simulink model "sampleModel153"  (R2021b)
settings: Solver=VariableStepAuto  StartTime=0.0  StopTime=10.0  RelTol=1e-3
undefined symbols (not defined in the file or in its folder): DiscIntNeverNeededParam
libraries: simulink x18, slpidlib x3
settings Model: Creator=user  LastModifiedBy=user

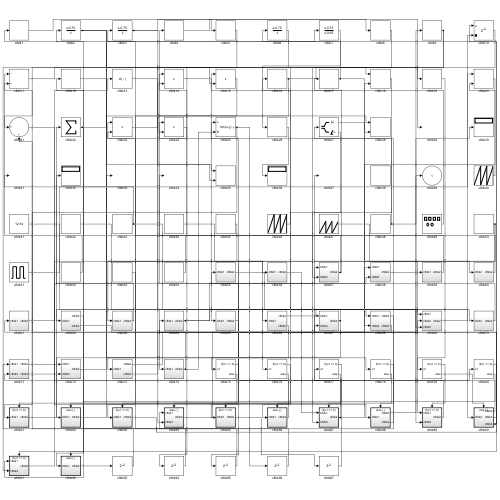
[thumbnail: Simulink's stored preview of the top-level diagram]
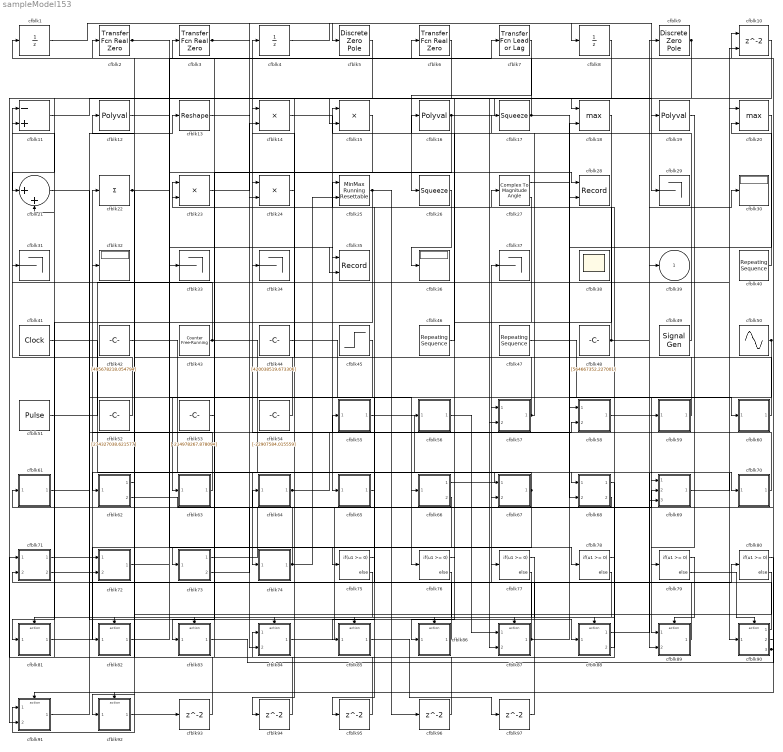
== system sampleModel153 ==
  cfblk1 : UnitDelay  HasFrameUpgradeWarning=on
  cfblk10 : Delay  ShowEnablePort=on  SampleTime=1
      settings: InputPortMap=u0,e6
  cfblk11 : Sum  Inputs=-+
  cfblk12 : Polyval  Coefs=[ +2.081618890e-019, -1.441693666e-014, +4.719686976e-010, -8.536869453e-006, +1.621573104e-001, -8.087801117e+001 ]
  cfblk13 : Reshape
  cfblk14 : Product
  cfblk15 : Product
  cfblk16 : Polyval  Coefs=[ +2.081618890e-019, -1.441693666e-014, +4.719686976e-010, -8.536869453e-006, +1.621573104e-001, -8.087801117e+001 ]
  cfblk17 : Squeeze
  cfblk18 : MinMax  Function=max  Inputs=2
  cfblk19 : Polyval  Coefs=[ +2.081618890e-019, -1.441693666e-014, +4.719686976e-010, -8.536869453e-006, +1.621573104e-001, -8.087801117e+001 ]
  cfblk2 : simulink/Discrete/Transfer Fcn Real Zero  ZeroZ=0.75  ICPrevInput=0.0  DoSatur=off
      settings: SourceProductBaseCode=SL
  cfblk20 : MinMax  Function=max  Inputs=2
  cfblk21 : Sum  Inputs=|++
  cfblk22 : Sum  Inputs=+
  cfblk23 : Product  Inputs=**
  cfblk24 : Product
  cfblk25 : simulink/Math Operations/MinMax Running Resettable  Function=min  vinit=0.0
  cfblk26 : Squeeze
  cfblk27 : ComplexToMagnitudeAngle
  cfblk28 : Record  FileSettingsInternal="{\"entries\":[{\"content\":{\"excelSettings\":{\"content\":{},\"type\":\"Streamout.ExcelSettings\"}},\"type\":\"Streamout.FileSettingStorage\",\"uuid\":\"2c212456-ffd4-42f7-90f6-1e0b846be94d\"}],\"packageUris\":[\"http://schema.mathworks.com/mf0/streamout_blocks/R2020a\"],\"version\":\"1.0\"}"  Layout=[1 1]  SignalsInternal="{\"entries\":[{\"content\":{\"signals\":[{\"content\":{\"blockPath\":[\"sampleModel153/cfblk28\"],\"channel\":[],\"dimensions\":[1],\"domain\":\"sampleModel153/cfblk28\",\"lineColor\":\"#a2142f\",\"plots\":[1],\"port\":1,\"sid\":[\"\"],\"signalID\":5763,\"signalName\":\"cfblk22\"},\"type\":\"RecordBlkView.Signal\",\"uuid\":\"cd0d1053-2d62-45ce-b0cb-306719bd41ca\"},{\"content\":{\"blockPath\":[\"sampleModel153/cfblk28\"],\"channel\":[],\"dimensions\":[1],\"domain\":\"sampleModel153/cfblk28\",\"lineColor\":\"#139fff\",\"plots\":[1],\"port\":2,\"sid\":[\"\"],\"signalID\":5767,\"signalName\":\"cfblk17\"},\"type\":\"RecordBlkView.Signal\",\"uuid\":\"0545e501-2640-4680-8aab-18a8a52ad5f1\"}]},\"type\":\"RecordBlkView.InputSignals\",\"uuid\":\"102c47a6-78df-4665-87ee-f45ed5971bb9\"}],\"packageUris\":[\"http://schema.mathworks.com/mf0/streamout_blocks/R2020a\"],\"version\":\"1.0\"}"  VisualizationBindings="{\"xyplotplugin\":{\"info\":[{\"series\":[{\"bindingParametersList\":[{\"parameter\":\"X-Axis\",\"signalID\":5763,\"signalName\":\"cfblk22\"},{\"parameter\":\"Y-Axis\",\"signalID\":5767,\"signalName\":\"cfblk17\"}],\"seriesID\":24473}],\"subplotID\":1}]}}"  CompatibilityTag=XY
  cfblk{29,31,33..34,37} (5 alike) : Terminator
  cfblk3 : simulink/Discrete/Transfer Fcn Real Zero  ZeroZ=0.75  ICPrevInput=0.0  DoSatur=off
      settings: SourceProductBaseCode=SL
  cfblk30 : Display
  cfblk32 : Display
  cfblk35 : Record  FileSettingsInternal="{\"entries\":[{\"content\":{\"excelSettings\":{\"content\":{},\"type\":\"Streamout.ExcelSettings\"}},\"type\":\"Streamout.FileSettingStorage\",\"uuid\":\"1263f3c2-cf19-49a5-a86e-01916edfd877\"}],\"packageUris\":[\"http://schema.mathworks.com/mf0/streamout_blocks/R2020a\"],\"version\":\"1.0\"}"  Layout=[1 1]  SignalsInternal="{\"entries\":[{\"content\":{\"signals\":[{\"content\":{\"blockPath\":[\"sampleModel153/cfblk35\"],\"channel\":[],\"dimensions\":[1],\"domain\":\"sampleModel153/cfblk35\",\"lineColor\":\"#a2142f\",\"plots\":[1],\"port\":1,\"sid\":[\"\"],\"signalID\":5771,\"signalName\":\"cfblk13\"},\"type\":\"RecordBlkView.Signal\",\"uuid\":\"12ff4bb5-13ec-4cb2-af01-71f94b166f3a\"},{\"content\":{\"blockPath\":[\"sampleModel153/cfblk35\"],\"channel\":[],\"dimensions\":[1],\"domain\":\"sampleModel153/cfblk35\",\"lineColor\":\"#139fff\",\"plots\":[1],\"port\":2,\"sid\":[\"\"],\"signalID\":5775,\"signalName\":\"cfblk12\"},\"type\":\"RecordBlkView.Signal\",\"uuid\":\"445a6bb3-1bb0-4b42-baa5-e16de1a42cbc\"}]},\"type\":\"RecordBlkView.InputSignals\",\"uuid\":\"a8e47f34-4e25-4855-b461-5707e96d08f3\"}],\"packageUris\":[\"http://schema.mathworks.com/mf0/streamout_blocks/R2020a\"],\"version\":\"1.0\"}"  VisualizationBindings="{\"xyplotplugin\":{\"info\":[{\"series\":[{\"bindingParametersList\":[{\"parameter\":\"X-Axis\",\"signalID\":5771,\"signalName\":\"cfblk13\"},{\"parameter\":\"Y-Axis\",\"signalID\":5775,\"signalName\":\"cfblk12\"}],\"seriesID\":38027}],\"subplotID\":1}]}}"  CompatibilityTag=XY
  cfblk36 : Display
  cfblk38 : Scope
      settings: Floating=on
  cfblk4 : UnitDelay  HasFrameUpgradeWarning=on
  cfblk40 : simulink/Sources/Repeating Sequence  rep_seq_t=[0 2]  rep_seq_y=[-482510888.410190, 936654599.798604]
  cfblk41 : DigitalClock
  cfblk42 : Constant  Value=[495678218.054794]  SampleTime=1
  cfblk43 : simulink/Sources/Counter Free-Running  NumBits=[26.000000]  tsamp=-1
  cfblk44 : Constant  Value=[420038519.673306]  SampleTime=1
  cfblk45 : Step  Time=[9.000000]  Before=[549406599.137464]  After=[-884570738.037617]  SampleTime=0
  cfblk46 : simulink/Sources/Repeating Sequence  rep_seq_t=[0 2]  rep_seq_y=[-989450428.873193, 779699657.139585]
  cfblk47 : simulink/Sources/Repeating Sequence  rep_seq_t=[0 2]  rep_seq_y=[-841389417.490251, -296508682.035901]
  cfblk48 : Constant  Value=[564667352.227001]  SampleTime=1
  cfblk49 : SignalGenerator  WaveForm=square  Amplitude=[-35189070.277397]
  cfblk5 : DiscreteZeroPole  Poles=[0 0.5]  Gain=1
  cfblk50 : Sin  Amplitude=[679153258.026251]  Bias=[71946484.496305]  SampleTime=0
  cfblk51 : DiscretePulseGenerator  PulseType=Time based  Amplitude=[-905572706.861220]  Period=[25399311.499519]  PulseWidth=5  PhaseDelay=[2.000000]
  cfblk52 : Constant  Value=[274327038.621577]  SampleTime=1
  cfblk53 : Constant  Value=[-214978267.878094]  SampleTime=1
  cfblk54 : Constant  Value=[-22907584.015559]  SampleTime=1
  cfblk55 : Subsystem
  cfblk56 : Subsystem
  cfblk57 : Subsystem
  cfblk58 : Subsystem
  cfblk59 : Subsystem
  cfblk6 : simulink/Discrete/Transfer Fcn Real Zero  ZeroZ=0.75  ICPrevInput=0.0  DoSatur=off
      settings: SourceProductBaseCode=SL
  cfblk60 : Subsystem
  cfblk61 : Subsystem
  cfblk62 : Subsystem
  cfblk63 : Subsystem
  cfblk64 : Subsystem
  cfblk65 : Subsystem
  cfblk66 : Subsystem
  cfblk67 : Subsystem
  cfblk68 : Subsystem
  cfblk69 : Subsystem
  cfblk7 : simulink/Discrete/Transfer Fcn Lead or Lag  PoleZ=0.95  ZeroZ=0.75  ICPrevOutput=0.0  ICPrevInput=0.0  DoSatur=off
      settings: SourceProductBaseCode=SL
  cfblk70 : Subsystem
  cfblk71 : Subsystem
  cfblk72 : Subsystem
  cfblk73 : Subsystem
  cfblk74 : Subsystem
  cfblk{75..80} (6 alike) : If  IfExpression=u1 >= 0  SampleTime=1
  cfblk8 : UnitDelay  HasFrameUpgradeWarning=on
  cfblk81 : Subsystem  TreatAsAtomicUnit=on
  cfblk82 : Subsystem  TreatAsAtomicUnit=on
  cfblk83 : Subsystem  TreatAsAtomicUnit=on
  cfblk84 : Subsystem  TreatAsAtomicUnit=on
  cfblk85 : Subsystem  TreatAsAtomicUnit=on
  cfblk86 : Subsystem  TreatAsAtomicUnit=on
  cfblk87 : Subsystem  TreatAsAtomicUnit=on
  cfblk88 : Subsystem  TreatAsAtomicUnit=on
  cfblk89 : Subsystem  TreatAsAtomicUnit=on
  cfblk9 : DiscreteZeroPole  Poles=[0 0.5]  Gain=1
  cfblk90 : Subsystem  TreatAsAtomicUnit=on
  cfblk91 : Subsystem  TreatAsAtomicUnit=on
  cfblk92 : Subsystem  TreatAsAtomicUnit=on
  cfblk{93..97} (5 alike) : Delay  SampleTime=1
  cfblk39 : Outport
  wires:
  cfblk16/1 -> cfblk18/1, cfblk24/2
  cfblk42/1 -> cfblk74/1(cfblk1)
  cfblk1/1 -> cfblk29/1
  cfblk7/1 -> cfblk26/1
  cfblk26/1 -> cfblk36/1
  cfblk56/1(cfblk2) -> cfblk87/1(cfblk1)
  cfblk5/1 -> cfblk23/1
  cfblk70/1(cfblk2) -> cfblk4/1
  cfblk22/1 -> cfblk28/1, cfblk92/1(cfblk1)
  cfblk68/1(cfblk2) -> cfblk84/1(cfblk1)
  cfblk47/1 -> cfblk89/1(cfblk1)
  cfblk48/1 -> cfblk9/1, cfblk27/1
  cfblk52/1 -> cfblk11/1
  cfblk44/1 -> cfblk76/1
  cfblk46/1 -> cfblk16/1
  cfblk8/1 -> cfblk66/1(cfblk1)
  cfblk3/1 -> cfblk5/1, cfblk69/3(cfblk5)
  cfblk15/1 -> cfblk83/1(cfblk1)
  cfblk88/1(cfblk2) -> cfblk30/1
  cfblk81/1(cfblk2) -> cfblk22/1
  cfblk66/1(cfblk2) -> cfblk69/1(cfblk1)
  cfblk62/1(cfblk2) -> cfblk91/1(cfblk1)
  cfblk87/1(cfblk2) -> cfblk18/2, cfblk71/2(cfblk3)
  cfblk14/1 -> cfblk65/1(cfblk1)
  cfblk63/1(cfblk2) -> cfblk32/1
  cfblk83/1(cfblk2) -> cfblk10/1
  cfblk57/1(cfblk2) -> cfblk12/1, cfblk17/1
  cfblk11/1 -> cfblk19/1
  cfblk90/1(cfblk2) -> cfblk37/1
  cfblk67/1(cfblk2) -> cfblk62/1(cfblk1), cfblk75/1
  cfblk21/1 -> cfblk88/1(cfblk1)
  cfblk51/1 -> cfblk10/2
  cfblk50/1 -> cfblk63/1(cfblk1), cfblk85/1(cfblk1)
  cfblk73/1(cfblk2) -> cfblk39/1
  cfblk41/1 -> cfblk89/2(cfblk5)
  cfblk72/1(cfblk2) -> cfblk33/1
  cfblk82/1(cfblk2) -> cfblk7/1
  cfblk19/1 -> cfblk79/1
  cfblk27/1 -> cfblk60/1(cfblk1)
  cfblk68/2(cfblk5) -> cfblk61/1(cfblk1)
  cfblk90/2(cfblk3) -> cfblk6/1
  cfblk10/1 -> cfblk91/2(cfblk4)
  cfblk43/1 -> cfblk31/1, cfblk90/1(cfblk1)
  cfblk88/2(cfblk3) -> cfblk24/1
  cfblk54/1 -> cfblk3/1
  cfblk64/1(cfblk2) -> cfblk68/1(cfblk1), cfblk58/2(cfblk5)
  cfblk55/1(cfblk2) -> cfblk70/1(cfblk1)
  cfblk73/2(cfblk5) -> cfblk67/1(cfblk1)
  cfblk66/2(cfblk5) -> cfblk82/1(cfblk1)
  cfblk6/1 -> cfblk21/1
  cfblk62/2(cfblk3) -> cfblk69/2(cfblk4)
  cfblk84/1(cfblk2) -> cfblk58/1(cfblk1)
  cfblk9/1 -> cfblk87/2(cfblk5), cfblk84/2(cfblk4)
  cfblk17/1 -> cfblk28/2, cfblk1/1
  cfblk60/1(cfblk2) -> cfblk14/1
  cfblk53/1 -> cfblk73/1(cfblk1)
  cfblk91/1(cfblk2) -> cfblk72/1(cfblk1)
  cfblk90/3(cfblk4) -> cfblk64/1(cfblk1), cfblk67/2(cfblk4)
  cfblk89/1(cfblk2) -> cfblk25/1
  cfblk4/1 -> cfblk8/1
  cfblk23/1 -> cfblk14/2
  cfblk45/1 -> cfblk72/2(cfblk5)
  cfblk18/1 -> cfblk86/1(cfblk1)
  cfblk49/1 -> cfblk15/1
  cfblk58/1(cfblk2) -> cfblk59/1(cfblk1)
  cfblk20/1 -> cfblk68/2(cfblk4)
  cfblk2/1 -> cfblk56/1(cfblk1), cfblk78/1, cfblk15/2
  cfblk69/1(cfblk2) -> cfblk20/1
  cfblk59/1(cfblk2) -> cfblk34/1
  cfblk13/1 -> cfblk35/1
  cfblk74/1(cfblk2) -> cfblk21/2, cfblk25/2
  cfblk61/1(cfblk2) -> cfblk57/1(cfblk1)
  cfblk40/1 -> cfblk20/2
  cfblk27/2 -> cfblk57/2(cfblk3)
  cfblk86/1(cfblk2) -> cfblk55/1(cfblk1)
  cfblk71/1(cfblk2) -> cfblk13/1
  cfblk25/1 -> cfblk81/1(cfblk1), cfblk96/1
  cfblk12/1 -> cfblk35/2
  cfblk71/2(cfblk4) -> cfblk80/1
  cfblk75/1 -> cfblk81/Action
  cfblk75/2 -> cfblk82/Action
  cfblk76/1 -> cfblk83/Action
  cfblk76/2 -> cfblk84/Action
  cfblk77/1 -> cfblk85/Action
  cfblk77/2 -> cfblk86/Action
  cfblk78/1 -> cfblk87/Action
  cfblk78/2 -> cfblk88/Action
  cfblk79/1 -> cfblk89/Action
  cfblk79/2 -> cfblk90/Action
  cfblk80/1 -> cfblk91/Action
  cfblk80/2 -> cfblk92/Action
  cfblk92/1(cfblk2) -> cfblk93/1
  cfblk93/1 -> cfblk71/1(cfblk1)
  cfblk24/1 -> cfblk94/1
  cfblk94/1 -> cfblk2/1
  cfblk65/1(cfblk2) -> cfblk95/1
  cfblk95/1 -> cfblk23/2
  cfblk96/1 -> cfblk11/2
  cfblk85/1(cfblk2) -> cfblk97/1
  cfblk97/1 -> cfblk77/1

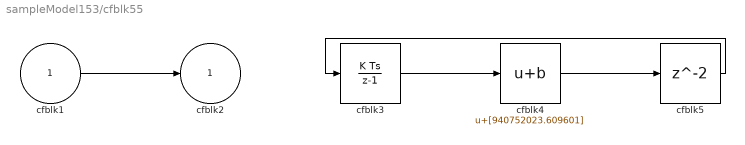
== system sampleModel153/cfblk55 ==
  cfblk1 : Inport
  cfblk3 : DiscreteIntegrator  ICPrevOutput=DiscIntNeverNeededParam  ICPrevScaledInput=DiscIntNeverNeededParam
  cfblk4 : Bias  Bias=[940752023.609601]
  cfblk5 : Delay  SampleTime=1
  cfblk2 : Outport
  wires:
  cfblk3/1 -> cfblk4/1
  cfblk1/1 -> cfblk2/1
  cfblk4/1 -> cfblk5/1
  cfblk5/1 -> cfblk3/1

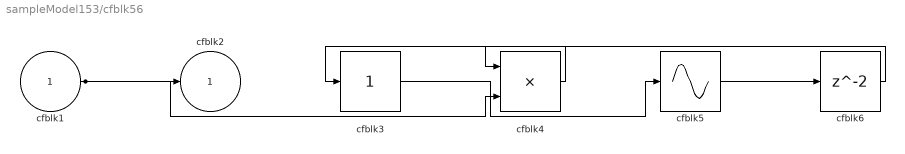
== system sampleModel153/cfblk56 ==
  cfblk1 : Inport
  cfblk3 : simulink/Math Operations/Slider Gain  gain=1  low=0  high=2
  cfblk4 : Product  Inputs=**
  cfblk5 : Sin  TimeSource=Use external signal  SampleTime=0
  cfblk6 : Delay  SampleTime=1
  cfblk2 : Outport
  wires:
  cfblk3/1 -> cfblk5/1
  cfblk1/1 -> cfblk4/2, cfblk2/1
  cfblk4/1 -> cfblk3/1
  cfblk5/1 -> cfblk6/1
  cfblk6/1 -> cfblk4/1

== system sampleModel153/cfblk57 ==
  cfblk1 : Inport
  cfblk3 : Inport  Port=2
  cfblk2 : Outport
  wires:
  cfblk3/1 -> cfblk2/1

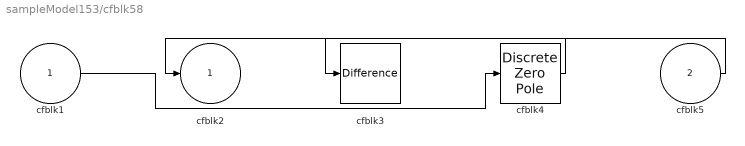
== system sampleModel153/cfblk58 ==
  cfblk1 : Inport
  cfblk5 : Inport  Port=2
  cfblk3 : simulink/Discrete/Difference  ICPrevInput=0.0  OutMin=[]  OutMax=[]  OutDataTypeStr=Inherit: Inherit via back propagation  OutDataType=fixdt(1, 16)  OutScaling=2^-10  DoSatur=off
  cfblk4 : DiscreteZeroPole  Poles=[0 0.5]  Gain=1
  cfblk2 : Outport
  wires:
  cfblk5/1 -> cfblk2/1
  cfblk1/1 -> cfblk4/1
  cfblk4/1 -> cfblk3/1

== system sampleModel153/cfblk59 ==
  cfblk1 : Inport
  cfblk3 : Product  Inputs=**
  cfblk2 : Outport
  wires:
  cfblk1/1 -> cfblk3/1, cfblk3/2
  cfblk3/1 -> cfblk2/1

== system sampleModel153/cfblk60 ==
  cfblk1 : Inport
  cfblk3 : Product
  cfblk2 : Outport
  wires:
  cfblk1/1 -> cfblk3/1, cfblk3/2
  cfblk3/1 -> cfblk2/1

== system sampleModel153/cfblk61 ==
  cfblk1 : Inport
  cfblk3 : Trigonometry
  cfblk2 : Outport
  wires:
  cfblk1/1 -> cfblk3/1
  cfblk3/1 -> cfblk2/1

== system sampleModel153/cfblk62 ==
  cfblk1 : Inport
  cfblk2 : Outport
  cfblk3 : Outport  Port=2
  wires:
  cfblk1/1 -> cfblk2/1, cfblk3/1

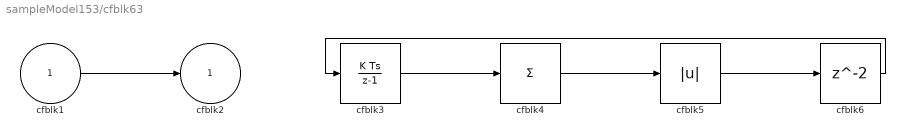
== system sampleModel153/cfblk63 ==
  cfblk1 : Inport
  cfblk3 : DiscreteIntegrator  ICPrevOutput=DiscIntNeverNeededParam  ICPrevScaledInput=DiscIntNeverNeededParam
  cfblk4 : Sum  Inputs=+
  cfblk5 : Abs
  cfblk6 : Delay  SampleTime=1
  cfblk2 : Outport
  wires:
  cfblk4/1 -> cfblk5/1
  cfblk3/1 -> cfblk4/1
  cfblk1/1 -> cfblk2/1
  cfblk5/1 -> cfblk6/1
  cfblk6/1 -> cfblk3/1

== system sampleModel153/cfblk64 ==
  cfblk1 : Inport
  cfblk3 : PermuteDimensions
  cfblk4 : Product
  cfblk2 : Outport
  wires:
  cfblk4/1 -> cfblk2/1
  cfblk1/1 -> cfblk3/1
  cfblk3/1 -> cfblk4/1, cfblk4/2

== system sampleModel153/cfblk65 ==
  cfblk1 : Inport
  cfblk3 : slpidlib/PID Controller  Controller=PID  Form=Parallel  TimeDomain=Discrete-time  UseExternalTs=off  SampleTime=1  IntegratorMethod=Forward Euler  FilterMethod=Forward Euler  ControllerParametersSource=internal  P=1  I=1  D=0  UseFilter=on  N=100  TunerSelectOption=Transfer Function Based (PID Tuner App)  InitialConditionSource=internal  InitialConditionForIntegrator=0  InitialConditionForFilter=0  DifferentiatorICPrevScaledInput=0  ExternalReset=none  TrackingMode=off  Kt=1  LimitOutput=off  SatLimitsSource=internal  UpperSaturationLimit=inf  LowerSaturationLimit=-inf  LinearizeAsGain=off  AntiWindupMode=none  Kb=1  POutMin=[]  POutMax=[]  IOutMin=[]  IOutMax=[]  DOutMin=[]  DOutMax=[]  NOutMin=[]  NOutMax=[]  SumOutMin=[]  SumOutMax=[]  SaturationOutMin=[]  SaturationOutMax=[]  PParamMin=[]  PParamMax=[]  IParamMin=[]  IParamMax=[]  DParamMin=[]  DParamMax=[]  NParamMin=[]  NParamMax=[]  KbParamMin=[]  KbParamMax=[]  KtParamMin=[]  KtParamMax=[]  KbOutMin=[]  KbOutMax=[]  KtOutMin=[]  KtOutMax=[]  IntegratorOutMin=[]  IntegratorOutMax=[]  FilterOutMin=[]  FilterOutMax=[]  SumI1OutMin=[]  SumI1OutMax=[]  SumI2OutMin=[]  SumI2OutMax=[]  SumI3OutMin=[]  SumI3OutMax=[]  SumI4OutMin=[]  SumI4OutMax=[]  SumDOutMin=[]  SumDOutMax=[]  DifferentiatorOutMin=[]  DifferentiatorOutMax=[]  FilterDiffOutCoefMin=[]  FilterDiffOutCoefMax=[]  ReciprocalOutMin=[]  ReciprocalOutMax=[]  SumDenOutMin=[]  SumDenOutMax=[]  SumNumOutMin=[]  SumNumOutMax=[]  DivideOutMin=[]  DivideOutMax=[]  UdiffTsProdOutMin=[]  UdiffTsProdOutMax=[]  NTsProdOutMin=[]  NTsProdOutMax=[]  UintegralTsProdOutMin=[]  UintegralTsProdOutMax=[]  UngainTsProdOutMin=[]  UngainTsProdOutMax=[]  IntegratorContinuousStateAttributes=''  IntegratorStateMustResolveToSignalObject=off  IntegratorRTWStateStorageClass=Auto  FilterContinuousStateAttributes=''  FilterStateMustResolveToSignalObject=off  FilterRTWStateStorageClass=Auto  ParallelPVariant=InternalParameters  IdealPVariant=Disabled  IVariant=InternalParameters  DVariant=InternalParameters  IntegratorVariant=Discrete  SatVariant=Disabled  AWVariant=Passthrough  PCopyVariant=Disabled  TRVariant=Disabled  FdbkBlocksVariant=Forward  IdealPFdbkVariant=Disabled  SatFdbkVariant=Disabled  DerivativeFilterVariant=ForwardEulerFilter  NVariant=InternalParameters  NCopyVariant=Disabled  FilterICVariant=InternalICsFilter  IntegratorICVariant=InternalICs  ExternalResetVariant=Disabled  TRSumVariant=Passthrough  SumFdbkVariant=Disabled  SumVariant=Sum_PID  TsampFilterVariant=InternalTs  TsampNgainVariant=Passthrough  TsampIntegralVariant=Passthrough  ExternalSaturationOutDataTypeStr=Inherit: Same as second input
  cfblk4 : UnaryMinus
  cfblk2 : Outport
  wires:
  cfblk4/1 -> cfblk3/1
  cfblk3/1 -> cfblk2/1
  cfblk1/1 -> cfblk4/1

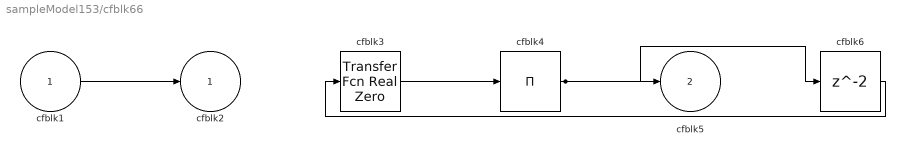
== system sampleModel153/cfblk66 ==
  cfblk1 : Inport
  cfblk3 : simulink/Discrete/Transfer Fcn Real Zero  ZeroZ=0.75  ICPrevInput=0.0  DoSatur=off
      settings: SourceProductBaseCode=SL
  cfblk4 : Product  Inputs=*
  cfblk6 : Delay  SampleTime=1
  cfblk2 : Outport
  cfblk5 : Outport  Port=2
  wires:
  cfblk4/1 -> cfblk5/1, cfblk6/1
  cfblk1/1 -> cfblk2/1
  cfblk3/1 -> cfblk4/1
  cfblk6/1 -> cfblk3/1

== system sampleModel153/cfblk67 ==
  cfblk1 : Inport
  cfblk4 : Inport  Port=2
  cfblk3 : Constant  Value=[-518749499.142794]  SampleTime=1
  cfblk2 : Outport
  wires:
  cfblk1/1 -> cfblk2/1

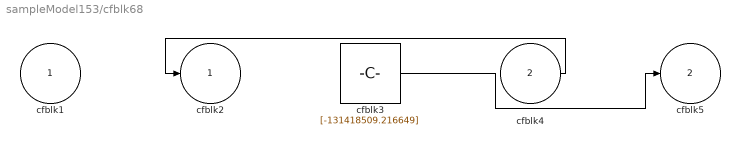
== system sampleModel153/cfblk68 ==
  cfblk1 : Inport
  cfblk4 : Inport  Port=2
  cfblk3 : Constant  Value=[-131418509.216649]  SampleTime=1
  cfblk2 : Outport
  cfblk5 : Outport  Port=2
  wires:
  cfblk4/1 -> cfblk2/1
  cfblk3/1 -> cfblk5/1

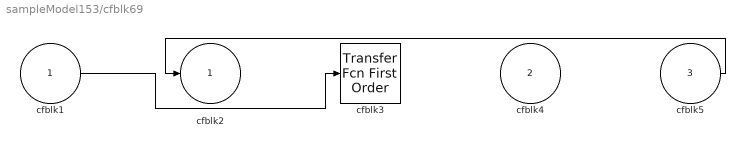
== system sampleModel153/cfblk69 ==
  cfblk1 : Inport
  cfblk4 : Inport  Port=2
  cfblk5 : Inport  Port=3
  cfblk3 : simulink/Discrete/Transfer Fcn First Order  PoleZ=0.95  ICPrevOutput=0.0  DoSatur=off
  cfblk2 : Outport
  wires:
  cfblk5/1 -> cfblk2/1
  cfblk1/1 -> cfblk3/1

== system sampleModel153/cfblk70 ==
  cfblk1 : Inport
  cfblk3 : simulink/Discrete/Transfer Fcn First Order  PoleZ=0.95  ICPrevOutput=0.0  DoSatur=off
  cfblk2 : Outport
  wires:
  cfblk3/1 -> cfblk2/1
  cfblk1/1 -> cfblk3/1

== system sampleModel153/cfblk71 ==
  cfblk1 : Inport
  cfblk3 : Inport  Port=2
  cfblk2 : Outport
  cfblk4 : Outport  Port=2
  wires:
  cfblk1/1 -> cfblk4/1
  cfblk3/1 -> cfblk2/1

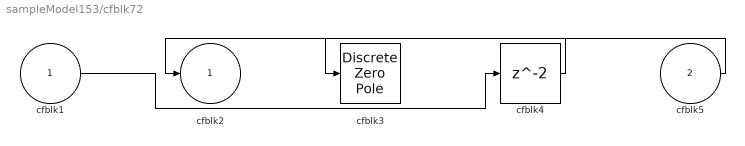
== system sampleModel153/cfblk72 ==
  cfblk1 : Inport
  cfblk5 : Inport  Port=2
  cfblk3 : DiscreteZeroPole  Poles=[0 0.5]  Gain=1
  cfblk4 : Delay  SampleTime=1
  cfblk2 : Outport
  wires:
  cfblk5/1 -> cfblk2/1
  cfblk1/1 -> cfblk4/1
  cfblk4/1 -> cfblk3/1

== system sampleModel153/cfblk73 ==
  cfblk1 : Inport
  cfblk3 : Sum  Inputs=|++
  cfblk4 : Constant  Value=[-692411394.663494]  SampleTime=1
  cfblk2 : Outport
  cfblk5 : Outport  Port=2
  wires:
  cfblk1/1 -> cfblk5/1, cfblk3/2
  cfblk4/1 -> cfblk3/1
  cfblk3/1 -> cfblk2/1

== system sampleModel153/cfblk74 ==
  cfblk1 : Inport
  cfblk3 : simulink/Discrete/Transfer Fcn Real Zero  ZeroZ=0.75  ICPrevInput=0.0  DoSatur=off
      settings: SourceProductBaseCode=SL
  cfblk4 : DiscreteFilter  SampleTime=1
  cfblk5 : UnitDelay  HasFrameUpgradeWarning=on
  cfblk2 : Outport
  wires:
  cfblk1/1 -> cfblk5/1, cfblk4/1
  cfblk3/1 -> cfblk2/1
  cfblk5/1 -> cfblk3/1

== system sampleModel153/cfblk81 ==
  cfblk1 : Inport
  Action Port : ActionPort  ActionPortLabel=if(u1 >= 0)
  cfblk3 : DiscreteStateSpace  SampleTime=-1
  cfblk2 : Outport
  wires:
  cfblk1/1 -> cfblk3/1
  cfblk3/1 -> cfblk2/1

== system sampleModel153/cfblk82 ==
  cfblk1 : Inport
  Action Port : ActionPort  ActionPortLabel=else
  cfblk3 : MinMax  Inputs=2
  cfblk4 : Constant  Value=[3125733.718125]  SampleTime=1
  cfblk2 : Outport
  wires:
  cfblk1/1 -> cfblk2/1, cfblk3/2
  cfblk4/1 -> cfblk3/1

== system sampleModel153/cfblk83 ==
  cfblk1 : Inport
  Action Port : ActionPort  ActionPortLabel=if(u1 >= 0)
  cfblk3 : simulink/Discrete/Transfer Fcn First Order  PoleZ=0.95  ICPrevOutput=0.0  DoSatur=off
  cfblk4 : slpidlib/PID Controller  Controller=PID  Form=Parallel  TimeDomain=Discrete-time  UseExternalTs=off  SampleTime=-1  IntegratorMethod=Forward Euler  FilterMethod=Forward Euler  ControllerParametersSource=internal  P=1  I=1  D=0  UseFilter=on  N=100  TunerSelectOption=Transfer Function Based (PID Tuner App)  InitialConditionSource=internal  InitialConditionForIntegrator=0  InitialConditionForFilter=0  DifferentiatorICPrevScaledInput=0  ExternalReset=none  TrackingMode=off  Kt=1  LimitOutput=off  SatLimitsSource=internal  UpperSaturationLimit=inf  LowerSaturationLimit=-inf  LinearizeAsGain=off  AntiWindupMode=none  Kb=1  POutMin=[]  POutMax=[]  IOutMin=[]  IOutMax=[]  DOutMin=[]  DOutMax=[]  NOutMin=[]  NOutMax=[]  SumOutMin=[]  SumOutMax=[]  SaturationOutMin=[]  SaturationOutMax=[]  PParamMin=[]  PParamMax=[]  IParamMin=[]  IParamMax=[]  DParamMin=[]  DParamMax=[]  NParamMin=[]  NParamMax=[]  KbParamMin=[]  KbParamMax=[]  KtParamMin=[]  KtParamMax=[]  KbOutMin=[]  KbOutMax=[]  KtOutMin=[]  KtOutMax=[]  IntegratorOutMin=[]  IntegratorOutMax=[]  FilterOutMin=[]  FilterOutMax=[]  SumI1OutMin=[]  SumI1OutMax=[]  SumI2OutMin=[]  SumI2OutMax=[]  SumI3OutMin=[]  SumI3OutMax=[]  SumI4OutMin=[]  SumI4OutMax=[]  SumDOutMin=[]  SumDOutMax=[]  DifferentiatorOutMin=[]  DifferentiatorOutMax=[]  FilterDiffOutCoefMin=[]  FilterDiffOutCoefMax=[]  ReciprocalOutMin=[]  ReciprocalOutMax=[]  SumDenOutMin=[]  SumDenOutMax=[]  SumNumOutMin=[]  SumNumOutMax=[]  DivideOutMin=[]  DivideOutMax=[]  UdiffTsProdOutMin=[]  UdiffTsProdOutMax=[]  NTsProdOutMin=[]  NTsProdOutMax=[]  UintegralTsProdOutMin=[]  UintegralTsProdOutMax=[]  UngainTsProdOutMin=[]  UngainTsProdOutMax=[]  IntegratorContinuousStateAttributes=''  IntegratorStateMustResolveToSignalObject=off  IntegratorRTWStateStorageClass=Auto  FilterContinuousStateAttributes=''  FilterStateMustResolveToSignalObject=off  FilterRTWStateStorageClass=Auto  ParallelPVariant=InternalParameters  IdealPVariant=Disabled  IVariant=InternalParameters  DVariant=InternalParameters  IntegratorVariant=Discrete  SatVariant=Disabled  AWVariant=Passthrough  PCopyVariant=Disabled  TRVariant=Disabled  FdbkBlocksVariant=Forward  IdealPFdbkVariant=Disabled  SatFdbkVariant=Disabled  DerivativeFilterVariant=ForwardEulerFilter  NVariant=InternalParameters  NCopyVariant=Disabled  FilterICVariant=InternalICsFilter  IntegratorICVariant=InternalICs  ExternalResetVariant=Disabled  TRSumVariant=Passthrough  SumFdbkVariant=Disabled  SumVariant=Sum_PID  TsampFilterVariant=InternalTs  TsampNgainVariant=Passthrough  TsampIntegralVariant=Passthrough  ExternalSaturationOutDataTypeStr=Inherit: Same as second input
  cfblk2 : Outport
  wires:
  cfblk1/1 -> cfblk3/1, cfblk4/1
  cfblk3/1 -> cfblk2/1

== system sampleModel153/cfblk84 ==
  cfblk1 : Inport
  cfblk4 : Inport  Port=2
  Action Port : ActionPort  ActionPortLabel=else
  cfblk3 : Sum  Inputs=+-
  cfblk2 : Outport
  wires:
  cfblk4/1 -> cfblk2/1
  cfblk1/1 -> cfblk3/1, cfblk3/2

== system sampleModel153/cfblk85 ==
  cfblk1 : Inport
  Action Port : ActionPort  ActionPortLabel=if(u1 >= 0)
  cfblk3 : simulink/Discrete/Transfer Fcn Lead or Lag  PoleZ=0.95  ZeroZ=0.75  ICPrevOutput=0.0  ICPrevInput=0.0  DoSatur=off
      settings: SourceProductBaseCode=SL
  cfblk2 : Outport
  wires:
  cfblk1/1 -> cfblk2/1, cfblk3/1

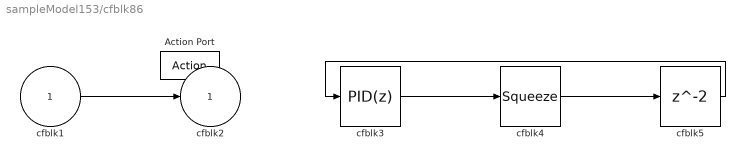
== system sampleModel153/cfblk86 ==
  cfblk1 : Inport
  Action Port : ActionPort  ActionPortLabel=else
  cfblk3 : slpidlib/PID Controller  Controller=PID  Form=Parallel  TimeDomain=Discrete-time  UseExternalTs=off  SampleTime=-1  IntegratorMethod=Forward Euler  FilterMethod=Forward Euler  ControllerParametersSource=internal  P=1  I=1  D=0  UseFilter=on  N=100  TunerSelectOption=Transfer Function Based (PID Tuner App)  InitialConditionSource=internal  InitialConditionForIntegrator=0  InitialConditionForFilter=0  DifferentiatorICPrevScaledInput=0  ExternalReset=none  TrackingMode=off  Kt=1  LimitOutput=off  SatLimitsSource=internal  UpperSaturationLimit=inf  LowerSaturationLimit=-inf  LinearizeAsGain=off  AntiWindupMode=none  Kb=1  POutMin=[]  POutMax=[]  IOutMin=[]  IOutMax=[]  DOutMin=[]  DOutMax=[]  NOutMin=[]  NOutMax=[]  SumOutMin=[]  SumOutMax=[]  SaturationOutMin=[]  SaturationOutMax=[]  PParamMin=[]  PParamMax=[]  IParamMin=[]  IParamMax=[]  DParamMin=[]  DParamMax=[]  NParamMin=[]  NParamMax=[]  KbParamMin=[]  KbParamMax=[]  KtParamMin=[]  KtParamMax=[]  KbOutMin=[]  KbOutMax=[]  KtOutMin=[]  KtOutMax=[]  IntegratorOutMin=[]  IntegratorOutMax=[]  FilterOutMin=[]  FilterOutMax=[]  SumI1OutMin=[]  SumI1OutMax=[]  SumI2OutMin=[]  SumI2OutMax=[]  SumI3OutMin=[]  SumI3OutMax=[]  SumI4OutMin=[]  SumI4OutMax=[]  SumDOutMin=[]  SumDOutMax=[]  DifferentiatorOutMin=[]  DifferentiatorOutMax=[]  FilterDiffOutCoefMin=[]  FilterDiffOutCoefMax=[]  ReciprocalOutMin=[]  ReciprocalOutMax=[]  SumDenOutMin=[]  SumDenOutMax=[]  SumNumOutMin=[]  SumNumOutMax=[]  DivideOutMin=[]  DivideOutMax=[]  UdiffTsProdOutMin=[]  UdiffTsProdOutMax=[]  NTsProdOutMin=[]  NTsProdOutMax=[]  UintegralTsProdOutMin=[]  UintegralTsProdOutMax=[]  UngainTsProdOutMin=[]  UngainTsProdOutMax=[]  IntegratorContinuousStateAttributes=''  IntegratorStateMustResolveToSignalObject=off  IntegratorRTWStateStorageClass=Auto  FilterContinuousStateAttributes=''  FilterStateMustResolveToSignalObject=off  FilterRTWStateStorageClass=Auto  ParallelPVariant=InternalParameters  IdealPVariant=Disabled  IVariant=InternalParameters  DVariant=InternalParameters  IntegratorVariant=Discrete  SatVariant=Disabled  AWVariant=Passthrough  PCopyVariant=Disabled  TRVariant=Disabled  FdbkBlocksVariant=Forward  IdealPFdbkVariant=Disabled  SatFdbkVariant=Disabled  DerivativeFilterVariant=ForwardEulerFilter  NVariant=InternalParameters  NCopyVariant=Disabled  FilterICVariant=InternalICsFilter  IntegratorICVariant=InternalICs  ExternalResetVariant=Disabled  TRSumVariant=Passthrough  SumFdbkVariant=Disabled  SumVariant=Sum_PID  TsampFilterVariant=InternalTs  TsampNgainVariant=Passthrough  TsampIntegralVariant=Passthrough  ExternalSaturationOutDataTypeStr=Inherit: Same as second input
  cfblk4 : Squeeze
  cfblk5 : Delay
  cfblk2 : Outport
  wires:
  cfblk3/1 -> cfblk4/1
  cfblk1/1 -> cfblk2/1
  cfblk4/1 -> cfblk5/1
  cfblk5/1 -> cfblk3/1

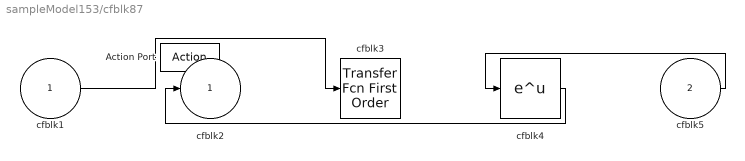
== system sampleModel153/cfblk87 ==
  cfblk1 : Inport
  cfblk5 : Inport  Port=2
  Action Port : ActionPort  ActionPortLabel=if(u1 >= 0)
  cfblk3 : simulink/Discrete/Transfer Fcn First Order  PoleZ=0.95  ICPrevOutput=0.0  DoSatur=off
  cfblk4 : Math  SaturateOnIntegerOverflow=on
  cfblk2 : Outport
  wires:
  cfblk5/1 -> cfblk4/1
  cfblk4/1 -> cfblk2/1
  cfblk1/1 -> cfblk3/1

== system sampleModel153/cfblk88 ==
  cfblk1 : Inport
  Action Port : ActionPort  ActionPortLabel=else
  cfblk2 : Outport
  cfblk3 : Outport  Port=2
  wires:
  cfblk1/1 -> cfblk3/1, cfblk2/1

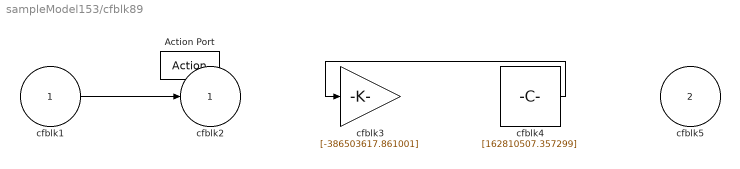
== system sampleModel153/cfblk89 ==
  cfblk1 : Inport
  cfblk5 : Inport  Port=2
  Action Port : ActionPort  ActionPortLabel=if(u1 >= 0)
  cfblk3 : Gain  Gain=[-386503617.861001]
  cfblk4 : Constant  Value=[162810507.357299]  SampleTime=1
  cfblk2 : Outport
  wires:
  cfblk1/1 -> cfblk2/1
  cfblk4/1 -> cfblk3/1

== system sampleModel153/cfblk90 ==
  cfblk1 : Inport
  Action Port : ActionPort  ActionPortLabel=else
  cfblk2 : Outport
  cfblk3 : Outport  Port=2
  cfblk4 : Outport  Port=3
  wires:
  cfblk1/1 -> cfblk4/1, cfblk3/1, cfblk2/1

== system sampleModel153/cfblk91 ==
  cfblk1 : Inport
  cfblk4 : Inport  Port=2
  Action Port : ActionPort  ActionPortLabel=if(u1 >= 0)
  cfblk3 : DiscreteFir
  cfblk2 : Outport
  wires:
  cfblk1/1 -> cfblk3/1
  cfblk3/1 -> cfblk2/1

== system sampleModel153/cfblk92 ==
  cfblk1 : Inport
  Action Port : ActionPort  ActionPortLabel=else
  cfblk3 : Math  Operator=hypot  SaturateOnIntegerOverflow=on
  cfblk2 : Outport
  wires:
  cfblk3/1 -> cfblk2/1
  cfblk1/1 -> cfblk3/1, cfblk3/2
